simulink model "untitled"  (R2016b)
settings: Solver=FixedStepAuto  StartTime=0.0  StopTime=0.2  FixedStep=0.00003  RelTol=1e-3
settings Model: Creator=Admin  LastModifiedBy=Admin

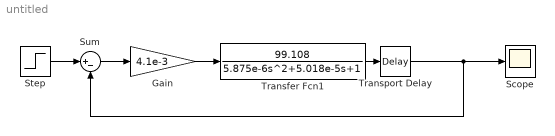
== system untitled ==
  Gain : Gain  Gain=4.1e-3
  Scope : Scope
  Step : Step  Time=0  SampleTime=0
  Sum : Sum  Inputs=|+-
  Transfer Fcn1 : TransferFcn  Numerator=[99.108]  Denominator=[5.875e-6 5.018e-5 1]
  Transport Delay : TransportDelay  DelayTime=1.25e-4
  wires:
  Step/1 -> Sum/1
  Sum/1 -> Gain/1
  Transport Delay/1 -> Sum/2, Scope/1
  Transfer Fcn1/1 -> Transport Delay/1
  Gain/1 -> Transfer Fcn1/1
